simulink model "VTOL_sim_Mk2"  (R2018a)
settings: Solver=VariableStepAuto  StartTime=0.0  StopTime=100  RelTol=1e-3
InitFcn:
  | vtol_param
StartFcn:
  | vtol_param
undefined symbols (not defined in the file or in its folder): P, PlotVtol
settings Model: Creator=sadam  LastModifiedBy=sadam

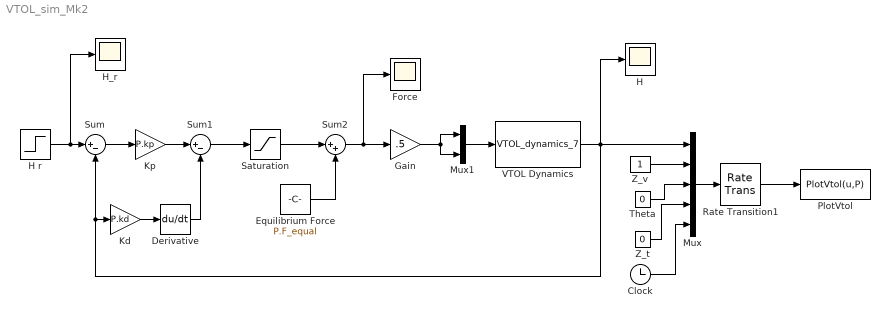
== system VTOL_sim_Mk2 ==
  Clock : Clock
  Derivative : Derivative
  Equilibrium Force : Constant  Value=P.F_equal
  Force : Scope
  Gain : Gain  Gain=.5
  H : Scope
  H r : Step  Time=3  After=4  SampleTime=0
  H_r : Scope
  Kd : Gain  Gain=P.kd
  Kp : Gain  Gain=P.kp
  Mux : Mux  Inputs=5
  Mux1 : Mux  Inputs=2
  "PlotVtol " : MATLABFcn  MATLABFcn=PlotVtol(u,P)  OutputDimensions=0
  Rate Transition1 : RateTransition  OutPortSampleTime=P.t_plot
  Saturation : Saturate  UpperLimit=P.Force_max  LowerLimit=-P.Force_max
  Sum : Sum  Inputs=|+-
  Sum1 : Sum  Inputs=|+-
  Sum2 : Sum  Inputs=|++
  Theta : Constant  Value=0
  VTOL Dynamics : S-Function  FunctionName=VTOL_dynamics_7  Parameters=P  SFunctionDeploymentMode=off  EnableBusSupport=off
  Z_t : Constant  Value=0
  Z_v : Constant
  wires:
  Sum/1 -> Kp/1
  Kd/1 -> Derivative/1
  Kp/1 -> Sum1/1
  Derivative/1 -> Sum1/2
  Mux/1 -> Rate Transition1/1
  VTOL Dynamics/1 -> H/1, Kd/1, Sum/2, Mux/1
  Gain/1 -> Mux1/2, Mux1/1
  H r/1 -> H_r/1, Sum/1
  Mux1/1 -> VTOL Dynamics/1
  Saturation/1 -> Sum2/1
  Sum2/1 -> Force/1, Gain/1
  Equilibrium Force/1 -> Sum2/2
  Sum1/1 -> Saturation/1
  Rate Transition1/1 -> "PlotVtol "/1
  Z_v/1 -> Mux/2
  Theta/1 -> Mux/3
  Z_t/1 -> Mux/4
  Clock/1 -> Mux/5
